simulink model "Fullcar_actuation_model"  (R2024b)
settings: Solver=VariableStepAuto  StartTime=0.0  StopTime=20  RelTol=1e-3
undefined symbols (not defined in the file): a, Af, b, Cf_sprung, Cf_unsprung, Cl, Cr_sprung, Cr_unsprung, g, I_PITCH, I_ROLL, Kf_sprung, Kf_unsprung, Kr_sprung, Kr_unsprung, M_sprung, Mf_unsprung, Mr_unsprung, rho, tw_front, tw_rear, v
settings Model: Creator=kanishka  LastModifiedBy=kanishka

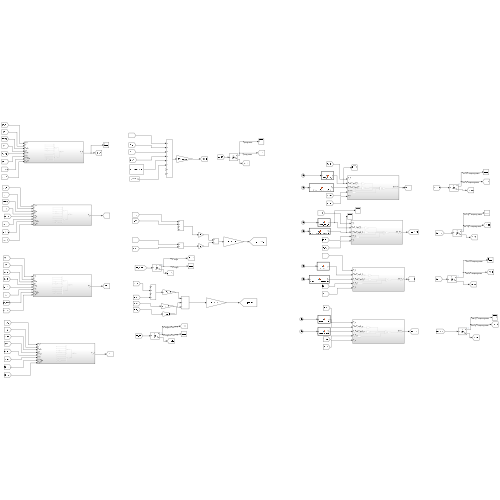
[thumbnail: Simulink's stored preview of the top-level diagram]
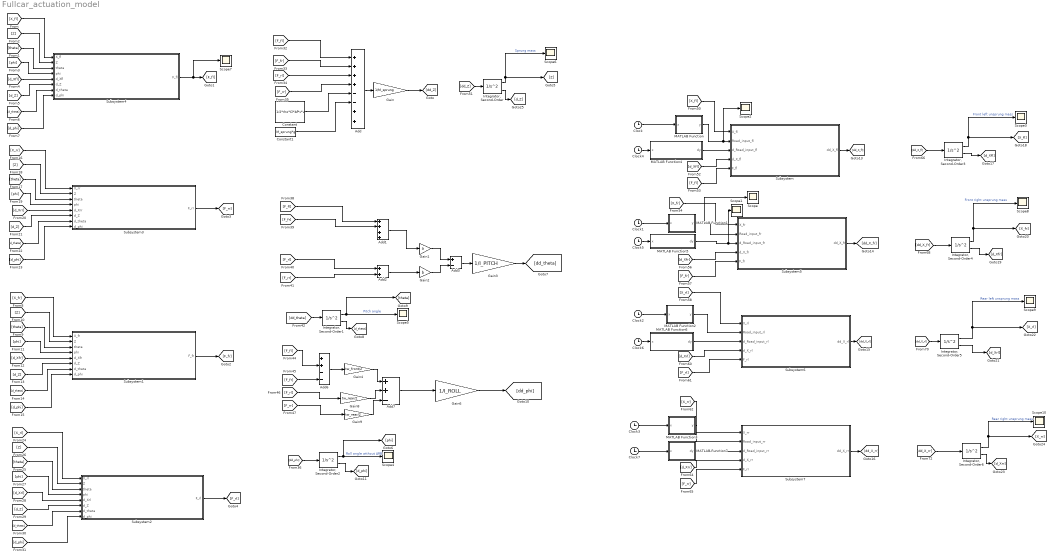
== system Fullcar_actuation_model ==
  Add : Sum  Inputs=++++--++
  Add1 : Sum  Inputs=++++
  Add2 : Sum
  Add3 : Sum  Inputs=+-
  Add6 : Sum  Inputs=++--
  Add7 : Sum  Inputs=++-
  Clock{,1..7} (8 alike) : Clock
  Constant : Constant  Value=1/2*rho*Cl*Af*v*v
  Constant1 : Constant  Value=M_sprung*g
  Gain : Gain  Gain=1/M_sprung
  Gain1 : Gain  Gain=a
  Gain2 : Gain  Gain=b
  Gain3 : Gain  Gain=1/I_PITCH
  Gain4 : Gain  Gain=tw_front/2
  Gain6 : Gain  Gain=1/I_ROLL
  Gain8 : Gain  Gain=tw_rear/2
  Gain9 : Gain  Gain=tw_rear/2
  Integrator, Second-Order{,1..6} (7 alike) : SecondOrderIntegrator
  MATLAB Function : MATLAB Function  TreatAsAtomicUnit=on
  MATLAB Function1 : MATLAB Function  TreatAsAtomicUnit=on
  MATLAB Function2 : MATLAB Function  TreatAsAtomicUnit=on
  MATLAB Function3 : MATLAB Function  TreatAsAtomicUnit=on
  MATLAB Function4 : MATLAB Function  TreatAsAtomicUnit=on
  MATLAB Function5 : MATLAB Function  TreatAsAtomicUnit=on
  MATLAB Function6 : MATLAB Function  TreatAsAtomicUnit=on
  MATLAB Function7 : MATLAB Function  TreatAsAtomicUnit=on
  Scope{,1..10} (11 alike) : Scope
  Subsystem : Subsystem
  Subsystem1 : Subsystem
  Subsystem2 : Subsystem
  Subsystem3 : Subsystem
  Subsystem4 : Subsystem
  Subsystem5 : Subsystem
  Subsystem6 : Subsystem
  Subsystem7 : Subsystem
  wires:
  Add/1 -> Gain/1
  Constant1/1 -> Add/6
  Constant/1 -> Add/5
  Gain/1 -> [dd_Z]
  Subsystem4/1(F_fl) -> Scope7/1, [F_fl]
  Subsystem1/1(F_fr) -> [F_fr]
  Subsystem3/1(F_rr) -> [F_rr]
  Subsystem2/1(F_rl) -> [F_rl]
  [X_fl] -> Subsystem4/1(X_fl)
  [Z] -> Subsystem4/2(Z)
  [theta] -> Subsystem4/3(theta)
  [phi] -> Subsystem4/4(phi)
  [d_Xfl] -> Subsystem4/5(d_Xfl)
  [d_Z] -> Subsystem4/6(d_Z)
  [d_theta] -> Subsystem4/7(d_theta)
  [d_phi] -> Subsystem4/8(d_phi)
  [d_Xfr] -> Subsystem1/5(d_Xfr)
  [d_theta] -> Subsystem1/7(d_theta)
  [phi] -> Subsystem1/4(phi)
  [Z] -> Subsystem1/2(Z)
  [d_phi] -> Subsystem1/8(d_phi)
  [X_fr] -> Subsystem1/1(X_fr)
  [theta] -> Subsystem1/3(theta)
  [d_Z] -> Subsystem1/6(d_Z)
  [d_Xrr] -> Subsystem3/5(d_Xrr)
  [d_theta] -> Subsystem3/7(d_theta)
  [phi] -> Subsystem3/4(phi)
  [Z] -> Subsystem3/2(Z)
  [d_phi] -> Subsystem3/8(d_phi)
  [X_rr] -> Subsystem3/1(X_rr)
  [theta] -> Subsystem3/3(theta)
  [d_Z] -> Subsystem3/6(d_Z)
  [phi] -> Subsystem2/4(phi)
  [d_theta] -> Subsystem2/7(d_theta)
  [d_Z] -> Subsystem2/6(d_Z)
  [X_rl] -> Subsystem2/1(X_rl)
  [d_Xrl] -> Subsystem2/5(d_Xrl)
  [d_phi] -> Subsystem2/8(d_phi)
  [Z] -> Subsystem2/2(Z)
  [theta] -> Subsystem2/3(theta)
  [F_fl] -> Add/1
  [F_fr] -> Add/2
  [F_rl] -> Add/3
  [F_rr] -> Add/4
  [F_fr] -> Add1/2
  [F_fl] -> Add1/1
  [F_rl] -> Add2/1
  [F_rr] -> Add2/2
  Add1/1 -> Gain1/1
  Add2/1 -> Gain2/1
  Gain1/1 -> Add3/1
  Gain2/1 -> Add3/2
  Add3/1 -> Gain3/1
  Gain3/1 -> [dd_theta]
  Gain6/1 -> [dd_phi]
  Add7/1 -> Gain6/1
  [X_fl] -> Subsystem/1(X_fl)
  MATLAB Function/1(y) -> Scope2/1, Subsystem/2(Road_input_fl)
  MATLAB Function4/1(dy) -> Subsystem/3(d_Road_input_fl)
  [d_Xfl] -> Subsystem/4(d_X_fl)
  [F_fl] -> Subsystem/5(F_fl)
  Clock/1 -> MATLAB Function/1(x)
  Subsystem/1(dd_X_fl) -> [dd_X_fl]
  Clock1/1 -> MATLAB Function1/1(x)
  [X_fr] -> Subsystem5/1(X_fr)
  MATLAB Function5/1(dy) -> Scope1/1, Subsystem5/3(d_Road_input_fr)
  [d_Xfr] -> Subsystem5/4(d_X_fr)
  [F_fr] -> Subsystem5/5(F_fr)
  Subsystem5/1(dd_X_fr) -> [dd_X_fr]
  Clock2/1 -> MATLAB Function2/1(x)
  [X_rl] -> Subsystem6/1(X_rl)
  MATLAB Function2/1(y) -> Subsystem6/2(Road_input_rl)
  MATLAB Function6/1(dy) -> Subsystem6/3(d_Road_input_rl)
  [d_Xrl] -> Subsystem6/4(d_X_rl)
  [F_rl] -> Subsystem6/5(F_rl)
  Subsystem6/1(dd_X_rl) -> [dd_X_rl]
  Clock3/1 -> MATLAB Function3/1(x)
  [X_rr] -> Subsystem7/1(X_rr)
  MATLAB Function3/1(y) -> Subsystem7/2(Road_input_rr)
  MATLAB Function7/1(dy) -> Subsystem7/3(d_Road_input_rr)
  [d_Xrr] -> Subsystem7/4(d_X_rr)
  [F_rr] -> Subsystem7/5(F_rr)
  Subsystem7/1(dd_X_rr) -> [dd_X_rr]
  [dd_X_fr] -> "Integrator, Second-Order4"/1
  "Integrator, Second-Order4"/2 -> [d_Xfr]
  [dd_X_rl] -> "Integrator, Second-Order5"/1
  "Integrator, Second-Order5"/2 -> [d_Xrl]
  [dd_X_rr] -> "Integrator, Second-Order6"/1
  Clock4/1 -> MATLAB Function4/1(x)
  Clock5/1 -> MATLAB Function5/1(x)
  Clock6/1 -> MATLAB Function6/1(x)
  Clock7/1 -> MATLAB Function7/1(x)
  MATLAB Function1/1(y) -> Scope/1, Subsystem5/2(Road_input_fr)
  [dd_Z] -> "Integrator, Second-Order"/1
  "Integrator, Second-Order"/2 -> [d_Z]
  "Integrator, Second-Order"/1 -> Scope6/1, [Z]  "Sprung mass"
  [dd_theta] -> "Integrator, Second-Order1"/1
  "Integrator, Second-Order1"/2 -> [d_theta]
  "Integrator, Second-Order1"/1 -> Scope5/1, [theta]  "Pitch angle"
  [dd_phi] -> "Integrator, Second-Order2"/1
  "Integrator, Second-Order2"/1 -> [phi], Scope4/1  "Roll angle without ARB"
  "Integrator, Second-Order2"/2 -> [d_phi]
  [dd_X_fl] -> "Integrator, Second-Order3"/1
  "Integrator, Second-Order3"/2 -> [d_Xfl]
  "Integrator, Second-Order3"/1 -> Scope3/1, [X_fl]  "Front left unsprung mass"
  "Integrator, Second-Order4"/1 -> [X_fr], Scope8/1  "Front right unsprung mass"
  "Integrator, Second-Order5"/1 -> Scope9/1, [X_rl]  "Rear left unsprung mass"
  "Integrator, Second-Order6"/2 -> [d_Xrr]
  "Integrator, Second-Order6"/1 -> [X_rr], Scope10/1  "Rear right unsprung mass"
  [F_rl] -> Gain8/1
  [F_rr] -> Gain9/1
  Gain4/1 -> Add7/1
  Gain8/1 -> Add7/2
  Gain9/1 -> Add7/3
  Add6/1 -> Gain4/1
  [F_fl] -> Add6/2
  [F_fr] -> Add6/4

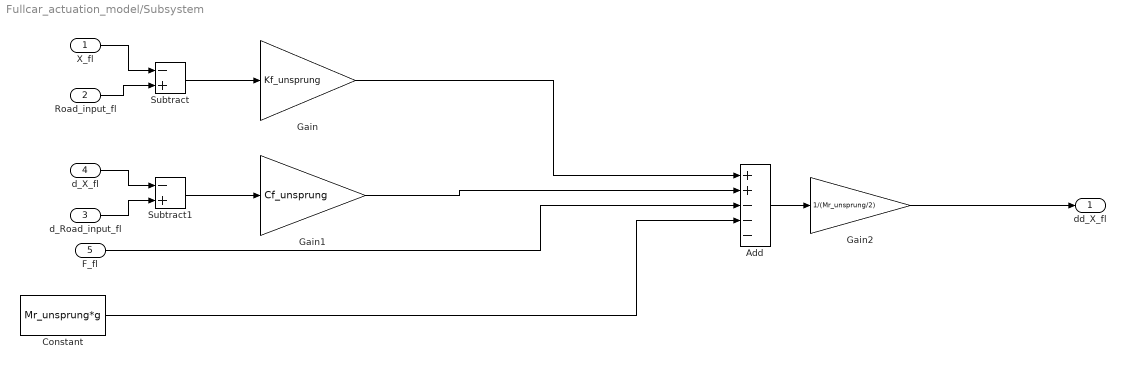
== system Fullcar_actuation_model/Subsystem ==
  X_fl : Inport
  Road_input_fl : Inport  Port=2
  d_Road_input_fl : Inport  Port=3
  d_X_fl : Inport  Port=4
  F_fl : Inport  Port=5
  Add : Sum  Inputs=++---
  Constant : Constant  Value=Mr_unsprung*g
  Gain : Gain  Gain=Kf_unsprung
  Gain1 : Gain  Gain=Cf_unsprung
  Gain2 : Gain  Gain=1/(Mr_unsprung/2)
  Subtract : Sum  Inputs=-+
  Subtract1 : Sum  Inputs=-+
  dd_X_fl : Outport
  wires:
  X_fl/1 -> Subtract/1
  Road_input_fl/1 -> Subtract/2
  Subtract/1 -> Gain/1
  d_Road_input_fl/1 -> Subtract1/2
  d_X_fl/1 -> Subtract1/1
  Subtract1/1 -> Gain1/1
  Gain/1 -> Add/1
  Gain1/1 -> Add/2
  F_fl/1 -> Add/3
  Constant/1 -> Add/4
  Add/1 -> Gain2/1
  Gain2/1 -> dd_X_fl/1

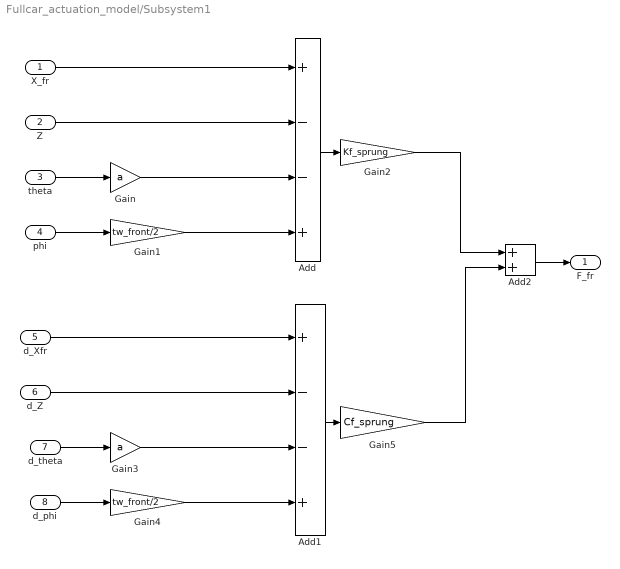
== system Fullcar_actuation_model/Subsystem1 ==
  X_fr : Inport
  Z : Inport  Port=2
  theta : Inport  Port=3
  phi : Inport  Port=4
  d_Xfr : Inport  Port=5
  d_Z : Inport  Port=6
  d_theta : Inport  Port=7
  d_phi : Inport  Port=8
  Add : Sum  Inputs=+--+
  Add1 : Sum  Inputs=+--+
  Add2 : Sum
  Gain : Gain  Gain=a
  Gain1 : Gain  Gain=tw_front/2
  Gain2 : Gain  Gain=Kf_sprung
  Gain3 : Gain  Gain=a
  Gain4 : Gain  Gain=tw_front/2
  Gain5 : Gain  Gain=Cf_sprung
  F_fr : Outport
  wires:
  Gain/1 -> Add/3
  Gain2/1 -> Add2/1
  Gain5/1 -> Add2/2
  Gain4/1 -> Add1/4
  Add/1 -> Gain2/1
  Gain1/1 -> Add/4
  Add2/1 -> F_fr/1
  Gain3/1 -> Add1/3
  Add1/1 -> Gain5/1
  theta/1 -> Gain/1
  d_theta/1 -> Gain3/1
  d_Xfr/1 -> Add1/1
  phi/1 -> Gain1/1
  d_phi/1 -> Gain4/1
  X_fr/1 -> Add/1
  d_Z/1 -> Add1/2
  Z/1 -> Add/2

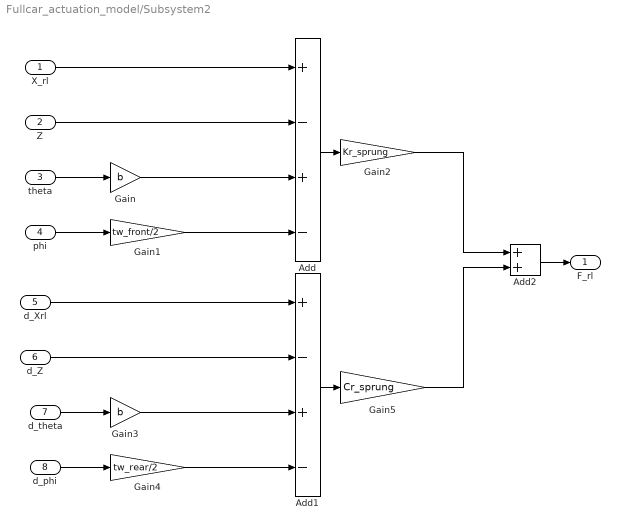
== system Fullcar_actuation_model/Subsystem2 ==
  X_rl : Inport
  Z : Inport  Port=2
  theta : Inport  Port=3
  phi : Inport  Port=4
  d_Xrl : Inport  Port=5
  d_Z : Inport  Port=6
  d_theta : Inport  Port=7
  d_phi : Inport  Port=8
  Add : Sum  Inputs=+-+-
  Add1 : Sum  Inputs=+-+-
  Add2 : Sum
  Gain : Gain  Gain=b
  Gain1 : Gain  Gain=tw_front/2
  Gain2 : Gain  Gain=Kr_sprung
  Gain3 : Gain  Gain=b
  Gain4 : Gain  Gain=tw_rear/2
  Gain5 : Gain  Gain=Cr_sprung
  F_rl : Outport
  wires:
  Gain4/1 -> Add1/4
  Gain/1 -> Add/3
  Gain3/1 -> Add1/3
  Gain5/1 -> Add2/2
  Gain2/1 -> Add2/1
  Add1/1 -> Gain5/1
  Add2/1 -> F_rl/1
  Add/1 -> Gain2/1
  Gain1/1 -> Add/4
  theta/1 -> Gain/1
  d_theta/1 -> Gain3/1
  d_Xrl/1 -> Add1/1
  phi/1 -> Gain1/1
  d_phi/1 -> Gain4/1
  X_rl/1 -> Add/1
  d_Z/1 -> Add1/2
  Z/1 -> Add/2

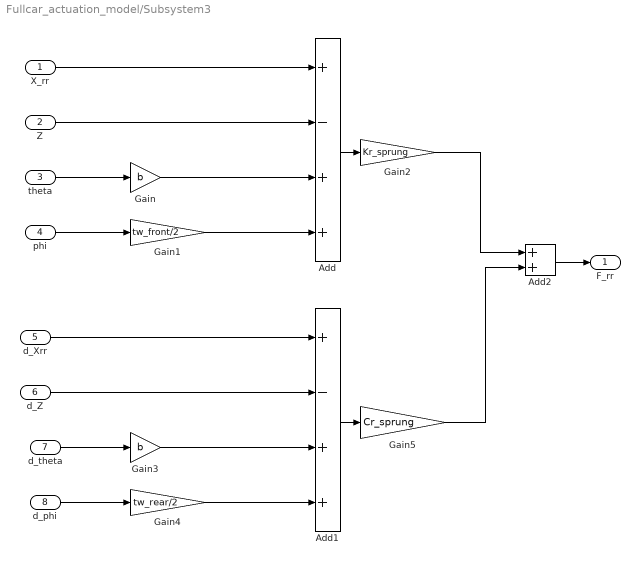
== system Fullcar_actuation_model/Subsystem3 ==
  X_rr : Inport
  Z : Inport  Port=2
  theta : Inport  Port=3
  phi : Inport  Port=4
  d_Xrr : Inport  Port=5
  d_Z : Inport  Port=6
  d_theta : Inport  Port=7
  d_phi : Inport  Port=8
  Add : Sum  Inputs=+-++
  Add1 : Sum  Inputs=+-++
  Add2 : Sum
  Gain : Gain  Gain=b
  Gain1 : Gain  Gain=tw_front/2
  Gain2 : Gain  Gain=Kr_sprung
  Gain3 : Gain  Gain=b
  Gain4 : Gain  Gain=tw_rear/2
  Gain5 : Gain  Gain=Cr_sprung
  F_rr : Outport
  wires:
  Gain/1 -> Add/3
  Gain5/1 -> Add2/2
  Gain3/1 -> Add1/3
  Add2/1 -> F_rr/1
  Gain1/1 -> Add/4
  Gain4/1 -> Add1/4
  Add1/1 -> Gain5/1
  Add/1 -> Gain2/1
  Gain2/1 -> Add2/1
  theta/1 -> Gain/1
  d_theta/1 -> Gain3/1
  d_Xrr/1 -> Add1/1
  phi/1 -> Gain1/1
  d_phi/1 -> Gain4/1
  X_rr/1 -> Add/1
  d_Z/1 -> Add1/2
  Z/1 -> Add/2

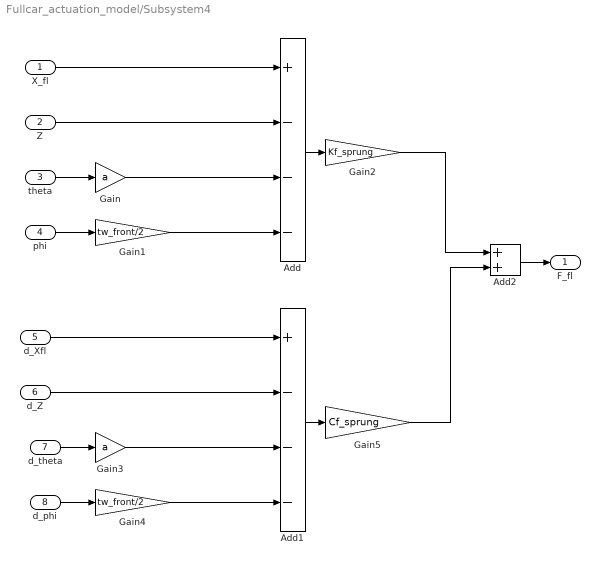
== system Fullcar_actuation_model/Subsystem4 ==
  X_fl : Inport
  Z : Inport  Port=2
  theta : Inport  Port=3
  phi : Inport  Port=4
  d_Xfl : Inport  Port=5
  d_Z : Inport  Port=6
  d_theta : Inport  Port=7
  d_phi : Inport  Port=8
  Add : Sum  Inputs=+---
  Add1 : Sum  Inputs=+---
  Add2 : Sum
  Gain : Gain  Gain=a
  Gain1 : Gain  Gain=tw_front/2
  Gain2 : Gain  Gain=Kf_sprung
  Gain3 : Gain  Gain=a
  Gain4 : Gain  Gain=tw_front/2
  Gain5 : Gain  Gain=Cf_sprung
  F_fl : Outport
  wires:
  Gain/1 -> Add/3
  Add/1 -> Gain2/1
  d_Xfl/1 -> Add1/1
  d_theta/1 -> Gain3/1
  Z/1 -> Add/2
  Gain3/1 -> Add1/3
  d_phi/1 -> Gain4/1
  Add1/1 -> Gain5/1
  Gain2/1 -> Add2/1
  Gain4/1 -> Add1/4
  Gain1/1 -> Add/4
  Gain5/1 -> Add2/2
  X_fl/1 -> Add/1
  Add2/1 -> F_fl/1
  theta/1 -> Gain/1
  phi/1 -> Gain1/1
  d_Z/1 -> Add1/2

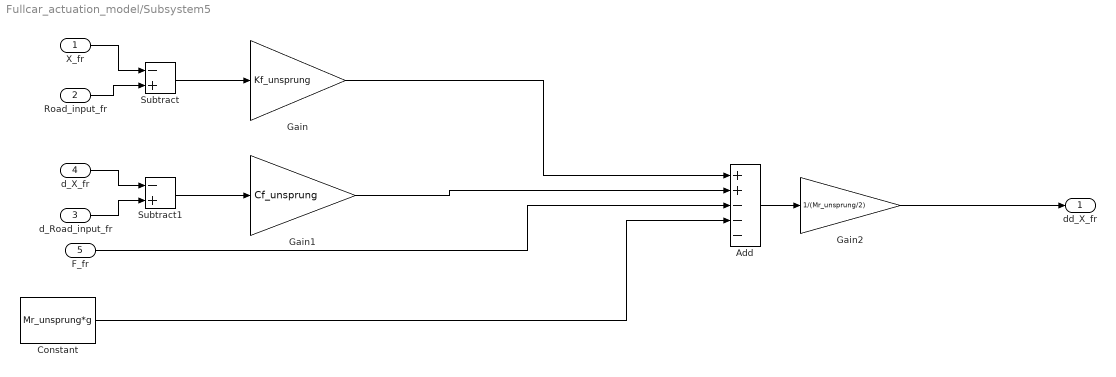
== system Fullcar_actuation_model/Subsystem5 ==
  X_fr : Inport
  Road_input_fr : Inport  Port=2
  d_Road_input_fr : Inport  Port=3
  d_X_fr : Inport  Port=4
  F_fr : Inport  Port=5
  Add : Sum  Inputs=++---
  Constant : Constant  Value=Mr_unsprung*g
  Gain : Gain  Gain=Kf_unsprung
  Gain1 : Gain  Gain=Cf_unsprung
  Gain2 : Gain  Gain=1/(Mr_unsprung/2)
  Subtract : Sum  Inputs=-+
  Subtract1 : Sum  Inputs=-+
  dd_X_fr : Outport
  wires:
  X_fr/1 -> Subtract/1
  Road_input_fr/1 -> Subtract/2
  Subtract/1 -> Gain/1
  d_Road_input_fr/1 -> Subtract1/2
  d_X_fr/1 -> Subtract1/1
  Subtract1/1 -> Gain1/1
  Gain/1 -> Add/1
  Gain1/1 -> Add/2
  F_fr/1 -> Add/3
  Constant/1 -> Add/4
  Add/1 -> Gain2/1
  Gain2/1 -> dd_X_fr/1

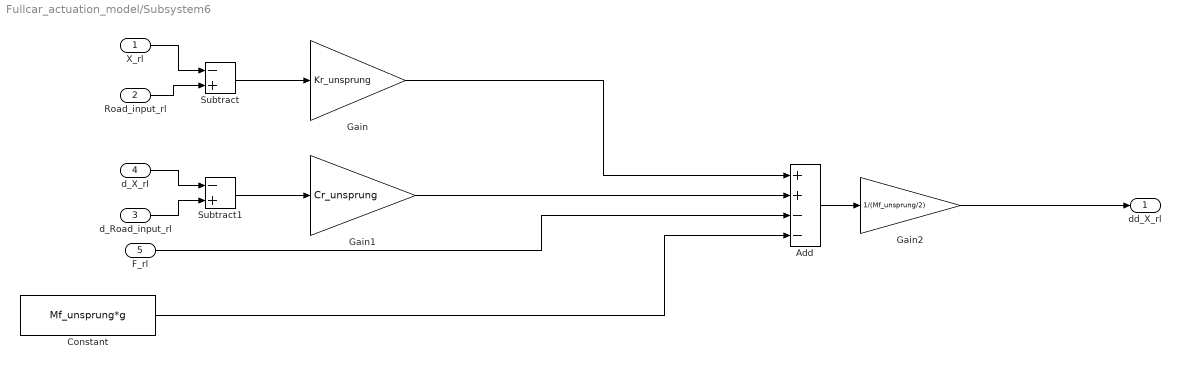
== system Fullcar_actuation_model/Subsystem6 ==
  X_rl : Inport
  Road_input_rl : Inport  Port=2
  d_Road_input_rl : Inport  Port=3
  d_X_rl : Inport  Port=4
  F_rl : Inport  Port=5
  Add : Sum  Inputs=++--
  Constant : Constant  Value=Mf_unsprung*g
  Gain : Gain  Gain=Kr_unsprung
  Gain1 : Gain  Gain=Cr_unsprung
  Gain2 : Gain  Gain=1/(Mf_unsprung/2)
  Subtract : Sum  Inputs=-+
  Subtract1 : Sum  Inputs=-+
  dd_X_rl : Outport
  wires:
  X_rl/1 -> Subtract/1
  Road_input_rl/1 -> Subtract/2
  Subtract/1 -> Gain/1
  d_Road_input_rl/1 -> Subtract1/2
  d_X_rl/1 -> Subtract1/1
  Subtract1/1 -> Gain1/1
  Gain/1 -> Add/1
  Gain1/1 -> Add/2
  F_rl/1 -> Add/3
  Constant/1 -> Add/4
  Add/1 -> Gain2/1
  Gain2/1 -> dd_X_rl/1

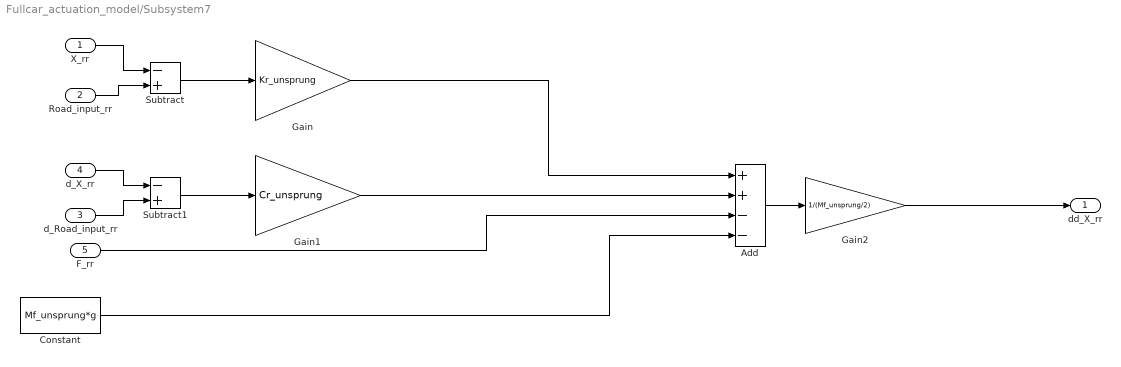
== system Fullcar_actuation_model/Subsystem7 ==
  X_rr : Inport
  Road_input_rr : Inport  Port=2
  d_Road_input_rr : Inport  Port=3
  d_X_rr : Inport  Port=4
  F_rr : Inport  Port=5
  Add : Sum  Inputs=++--
  Constant : Constant  Value=Mf_unsprung*g
  Gain : Gain  Gain=Kr_unsprung
  Gain1 : Gain  Gain=Cr_unsprung
  Gain2 : Gain  Gain=1/(Mf_unsprung/2)
  Subtract : Sum  Inputs=-+
  Subtract1 : Sum  Inputs=-+
  dd_X_rr : Outport
  wires:
  X_rr/1 -> Subtract/1
  Road_input_rr/1 -> Subtract/2
  Subtract/1 -> Gain/1
  d_Road_input_rr/1 -> Subtract1/2
  d_X_rr/1 -> Subtract1/1
  Subtract1/1 -> Gain1/1
  Gain/1 -> Add/1
  Gain1/1 -> Add/2
  F_rr/1 -> Add/3
  Constant/1 -> Add/4
  Add/1 -> Gain2/1
  Gain2/1 -> dd_X_rr/1

== matlab function Fullcar_actuation_model/MATLAB Function ==
  data: x input; y output
function y =Road_input_fl(x)

amplitude = 0.05;     
wavelength = 0.6;      
                
if x >= 0 && x <= wavelength/2
    y = amplitude * sin((2*pi * x) / wavelength);
else
    y = 0;
end
end

== matlab function Fullcar_actuation_model/MATLAB Function2 ==
  data: x input; y output
function y = Road_input_rl(x)
amplitude = 0.05;     
wavelength = 0.6;      
               
L = 1.53/2;             

if x >= L && x <=L+(wavelength/2)
    y = amplitude * sin(2*pi * (x-L) / wavelength);
else
    y = 0;
end
end

== matlab function Fullcar_actuation_model/MATLAB Function3 ==
  data: x input; y output
function y = Road_input_rr(x)
amplitude = 0.1;     
wavelength = 0.6;      
               
L = 1.53/2;             
if x >= L && x <=L+(wavelength/2)
    y = amplitude * sin(2*pi * (x-L) / wavelength);
else
    y = 0;
end
end

== matlab function Fullcar_actuation_model/MATLAB Function4 ==
  data: x input; dy output
function dy = Road_input_fl_derivative(x)

amplitude = 0.05;     % Amplitude of the sine wave
wavelength = 0.6;     % Wavelength (m)

% Derivative of half sine wave profile for 0 <= x <= 0.3
if x >= 0 && x <= wavelength/2
    dy = amplitude * (2*pi / wavelength) * cos((2*pi * x) / wavelength);
else
    dy = 0;
end

== matlab function Fullcar_actuation_model/MATLAB Function5 ==
  data: x input; dy output
function dy = Road_input_fr_derivative(x)

amplitude = 0.1;      % Amplitude of the sine wave
wavelength = 0.6;     % Wavelength of the sine wave

% Derivative of the half-sine wave for 0 <= x <= 0.3
if x >= 0 && x <= wavelength/2
    dy = amplitude * (2*pi / wavelength) * cos((2*pi * x) / wavelength);
else
    dy = 0;
end
end

== matlab function Fullcar_actuation_model/MATLAB Function6 ==
  data: x input; dy output
function dy = Road_input_rl_derivative(x)
amplitude = 0.05;
wavelength = 0.6;
L = 1.53 / 2;

if x >= L && x <= L + (wavelength / 2)
    dy = amplitude * (2*pi / wavelength) * cos(2 * pi * (x - L) / wavelength);
else
    dy = 0;
end
end

== matlab function Fullcar_actuation_model/MATLAB Function7 ==
  data: x input; dy output
function dy = Road_input_rr_derivative(x)
amplitude = 0.1;
wavelength = 0.6;
L = 1.53 / 2;

if x >= L && x <= L + (wavelength / 2)
    dy = amplitude * (2*pi / wavelength) * cos(2 * pi * (x - L) / wavelength);
else
    dy = 0;
end
end

== matlab function Fullcar_actuation_model/MATLAB Function1 ==
  data: x input; y output
function y = Road_input_fr(x)

amplitude = 0.1;     
wavelength = 0.6;      
               
if x >= 0 && x <= wavelength/2
    y = amplitude * sin((2*pi * x) / wavelength);
else
    y = 0;
end
end
